simulink model "wood_berry"  (R2021a)
settings: Solver=VariableStepAuto  StartTime=0.0  StopTime=100  RelTol=1e-3
values from neighbouring files (symbols this model uses):
  A = [-2 0; 1 -3]    [sistemas_lineares.m]    (also in wandb.m = sys.A)
  B = [0.5; 0]    [sistemas_lineares.m]    (also in wandb.m = sys.B)
  C = [0 1]    [sistemas_lineares.m]    (also in wandb.m = sys.C)
  D = 0    [sistemas_lineares.m]    (also in wandb.m = sys.D)
libraries: cstblocks x2
settings Model: Creator=Aula  LastModifiedBy=Aula

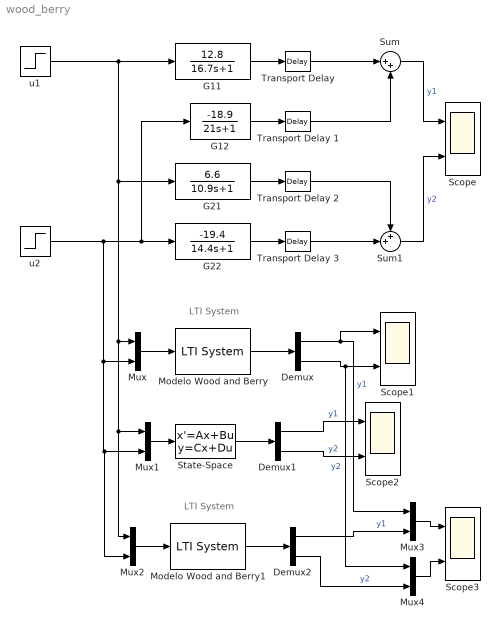
== system wood_berry ==
  note: LTI System
  note: LTI System
  Demux : Demux  Outputs=2
  Demux1 : Demux  Outputs=2
  Demux2 : Demux  Outputs=2
  G11 : TransferFcn  Numerator=[12.8]  Denominator=[16.7 1]
  G12 : TransferFcn  Numerator=[-18.9]  Denominator=[21 1]
  G21 : TransferFcn  Numerator=[6.6]  Denominator=[10.9 1]
  G22 : TransferFcn  Numerator=[-19.4]  Denominator=[14.4 1]
  Modelo Wood and Berry : cstblocks/LTI System  sys=G  IC=[]
  Modelo Wood and Berry1 : cstblocks/LTI System  sys=Gz  IC=[]
  Mux{,1..4} (5 alike) : Mux  Inputs=2
  Scope{,1..3} (4 alike) : Scope  NumInputPorts=2
  "State-Space " : StateSpace  A=A  B=B  C=C  D=D  InitialCondition=0
  Sum : Sum  Inputs=|++
  Sum1 : Sum  Inputs=++|
  "Transport Delay " : TransportDelay
  Transport Delay 1 : TransportDelay  DelayTime=3
  Transport Delay 2 : TransportDelay  DelayTime=7
  Transport Delay 3 : TransportDelay  DelayTime=3
  u1 : Step  Time=10  SampleTime=0
  u2 : Step  Time=50  SampleTime=0
  wires:
  G11/1 -> "Transport Delay "/1
  G12/1 -> Transport Delay 1/1
  G21/1 -> Transport Delay 2/1
  G22/1 -> Transport Delay 3/1
  Transport Delay 3/1 -> Sum1/2
  Transport Delay 2/1 -> Sum1/1
  Transport Delay 1/1 -> Sum/2
  "Transport Delay "/1 -> Sum/1
  Sum/1 -> Scope/1  "y1"
  Sum1/1 -> Scope/2  "y2"
  Mux/1 -> Modelo Wood and Berry/1
  Modelo Wood and Berry/1 -> Demux/1
  Demux/1 -> Mux3/1, Scope1/1  "y1"
  Demux/2 -> Mux4/1, Scope1/2  "y2"
  Mux1/1 -> "State-Space "/1
  "State-Space "/1 -> Demux1/1
  Demux1/1 -> Scope2/1  "y1"
  Demux1/2 -> Scope2/2  "y2"
  Modelo Wood and Berry1/1 -> Demux2/1
  Mux2/1 -> Modelo Wood and Berry1/1
  u2/1 -> Mux2/2, Mux1/2, Mux/2, G12/1, G22/1
  u1/1 -> Mux2/1, Mux1/1, Mux/1, G21/1, G11/1
  Mux3/1 -> Scope3/1
  Mux4/1 -> Scope3/2
  Demux2/1 -> Mux3/2  "y1"
  Demux2/2 -> Mux4/2  "y2"
